simulink model "Hexa_CAD_ANSFT_Sim"  (R2024b)
settings: Solver=ode4  StartTime=0.0  StopTime=8  FixedStep=0.01  RelTol=1e-3
model workspace (MAT data in the model file):
  hover_2m = [0  0  0  0  0  0; 0  0  0  0  0  0; 2  2  2  2  2  2; 0  0  0  0  0  0; 0  0  0  0  0  0; 0  0  0  0  0  0]
  square = [0  0  0  0  0  0; 0  0  0  0  0  0; 2.5  2.5  2.5  2.5  2.5  0; 0  0  0  0  0  0; 0  0  0  0  0  0; 0  0  0  0  0  0]
  tf = Simulink.Parameter
  tf.Value = 60
  tf.Complexity = 'real'
  tf.Dimensions = [1 1]
  tf.DataType = 'auto'
  tray0 = [0  0.2  0  0  0  0; 0  0.15  0  0  0  0; 0  2  2  2  2  0; 0  0  0  0  0  0; 0  0  0  0  0  0; 0  0  0  0  0  0]
  tray1 = [0  0  0  0  0  0; 0  0  0  0  0  0; 0  5  2.5  5  2.5  0; 0  0  0  0  0  0; 0  0  0  0  0  0; 0  0  0  0  0  0]
  tray2 = [0  2  2  -2  -2  0; 0  0  -2  -2  2  0; 0  5  2.5  5  2.5  0; 0  0  0  0  0  0; 0  0  0  0  0  0; 0  0  0  0  0  0]
  tray3 = [0  2  2  -2  -2  0; 0  0  -2  -2  2  0; 0  5  2.5  5  2.5  0; 0  0  0  0  0  0; 0  0  0  0  0  0; 0  0  0.785  1.042  0.785  0]
  tray4 = [0  2  2  -2  -2  0; 0  0  -2  -2  2  0; 0  5  2.5  5  2.5  0; 0  0.15  0.15  0.15  0.15  0; 0  0  0  0  0  0; 0  0  0.785  1.57  0.785  0]
  tray5 = [0  0  0  0  0  0; 0  0  0  0  0  0; 0  5  2.5  5  2.5  0; 0  0.15  0.15  0  0  0; 0  0  0.15  0.15  0  0; 0  0  0  0  0  0]
  tray_yaw = [0  0  0  0  0  0; 0  0  0  0  0  0; 0  5  2.5  5  2.5  0; 0  0  0  0  0  0; 0  0  0  0  0  0; 0  0  0.785  1.57  0.785  0]
undefined symbols (not defined in the file or in its folder): F, Light, MIL, smiData, X, Y, Z
libraries: sm_lib x238, nesl_utility x29, dspobslib x7, simulink x3, sharedtransform x2, robotcorelib x1, aerolibwind2 x1
(part 1 of 6)
settings Model: Creator=Jorge  LastModifiedBy=danyy
settings DataIOCC: ReturnWorkspaceOutputs=off
settings OptimizationCC: ReuseModelBlockBuffer=off
settings DebuggingCC: UnconnectedInputMsg=warning  UnconnectedOutputMsg=warning  UnconnectedLineMsg=warning
settings ModelReferenceCC: EnableRefExpFcnMdlSchedulingChecks=on
settings RTWCC: GPUComputeCapability=3.5  DLArmComputeVersion=19.05

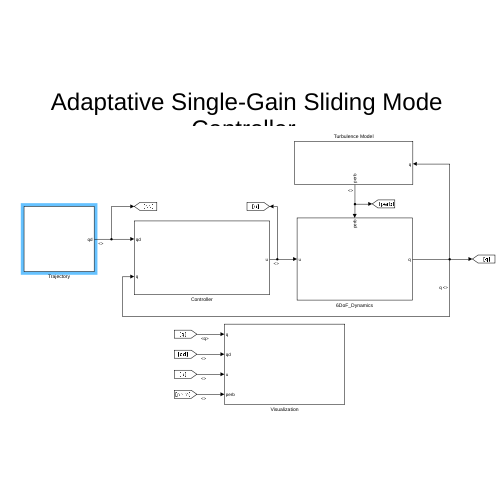
[thumbnail: Simulink's stored preview of the top-level diagram]
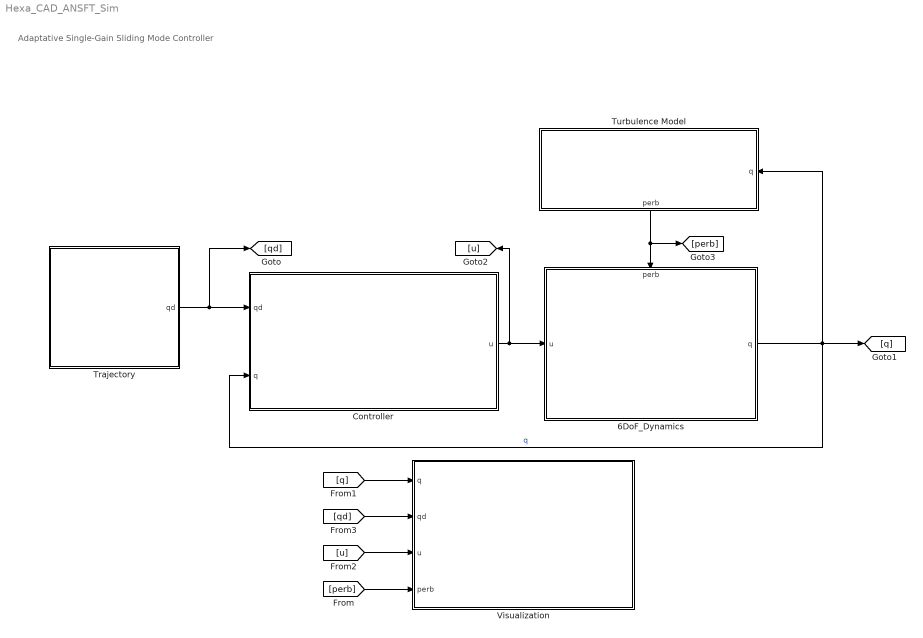
== system Hexa_CAD_ANSFT_Sim ==
  note: Adaptative Single-Gain Sliding Mode Controller
  6DoF_Dynamics : Subsystem
      settings: PortSchema="{\"entries\":[{\"content\":{\"sides\":[{\"content\":{\"connectorIds\":[\"In1\"]},\"type\":\"ConnectorPlacement.EquallySpacedRectSide\",\"uuid\":\"d79ec49c-5563-41e0-ac59-6e897bc19fda\"},{\"content\":{\"connectorIds\":[\"Out1\"],\"side\":\"RIGHT\"},\"type\":\"ConnectorPlacement.EquallySpacedRectSide\",\"uuid\":\"1255043e-c90e-4bae-9fb4-4fa06f36f53e\"},{\"content\":{\"connectorIds\":[\"In2\"],\"side\":\"TOP\"},\"type\":\"ConnectorPlacement.EquallySpacedRectSide\",\"uuid\":\"823ada36-3f22-4ee3-87a1-180276f622bc\"}]},\"type\":\"ConnectorPlacement.EquallySpacedConnector\",\"uuid\":\"7403b609-b333-4977-a854-ed7a71f74338\"}],\"packageUris\":[\"http://schema.mathworks.com/mf0/Connector/R2020b\"],\"version\":\"1.0\"}"
  Controller : Subsystem
  Trajectory : Subsystem
  Turbulence Model : Subsystem
      settings: PortSchema="{\"entries\":[{\"content\":{\"sides\":[{\"content\":{},\"type\":\"ConnectorPlacement.EquallySpacedRectSide\",\"uuid\":\"f78b09a1-2be7-4ada-a431-40e3e9754158\"},{\"content\":{\"connectorIds\":[\"In1\"],\"side\":\"RIGHT\"},\"type\":\"ConnectorPlacement.EquallySpacedRectSide\",\"uuid\":\"90af6136-accc-442b-9679-ef2510f8cfdd\"},{\"content\":{\"side\":\"TOP\"},\"type\":\"ConnectorPlacement.EquallySpacedRectSide\",\"uuid\":\"ed3143b1-02fd-44b4-8f22-c95c41bbcf7f\"},{\"content\":{\"connectorIds\":[\"Out1\"],\"side\":\"BOTTOM\"},\"type\":\"ConnectorPlacement.EquallySpacedRectSide\",\"uuid\":\"715dd93d-905b-40a3-aeb3-61c6c8d9767d\"}]},\"type\":\"ConnectorPlacement.EquallySpacedConnector\",\"uuid\":\"95dc4bc2-a941-4378-8d0a-e3a54b47d1ac\"}],\"packageUris\":[\"http://schema.mathworks.com/mf0/Connector/R2020b\"],\"version\":\"1.0\"}"
  Visualization : Subsystem
  wires:
  Trajectory/1(qd) -> [qd], Controller/1(qd)
  Controller/1(u) -> [u], 6DoF_Dynamics/1(u)
  6DoF_Dynamics/1(q) -> Turbulence Model/1(q), [q], Controller/2(q)  "q"
  Turbulence Model/1(perb) -> 6DoF_Dynamics/2(perb), [perb]
  [q] -> Visualization/1(q)
  [qd] -> Visualization/2(qd)
  [perb] -> Visualization/4(perb)
  [u] -> Visualization/3(u)

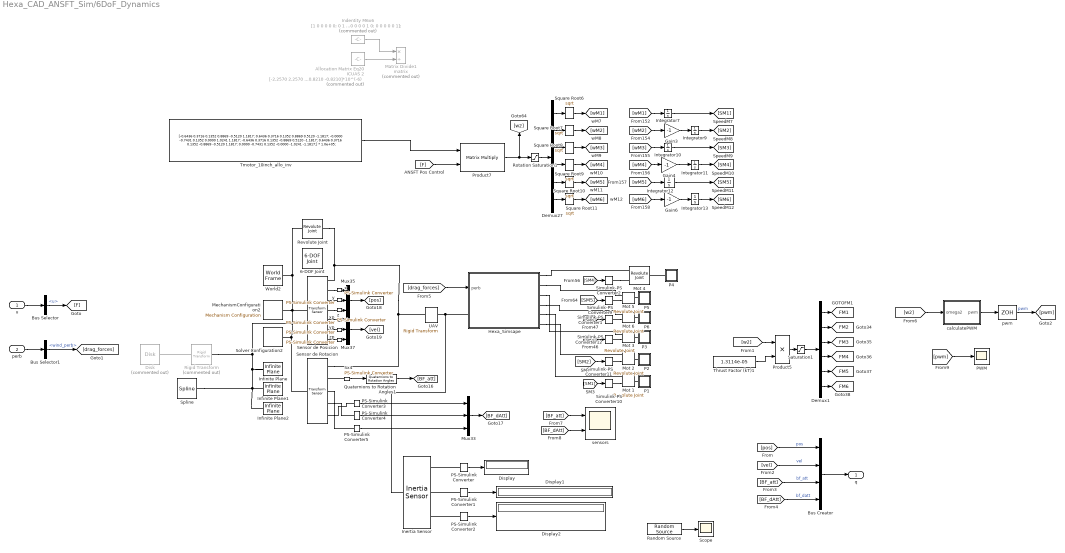
== system Hexa_CAD_ANSFT_Sim/6DoF_Dynamics ==
  u : Inport
  perb : Inport  Port=2
  6-DOF Joint : sm_lib/Joints/6-DOF Joint  JointMode=Normal  CompositeWrenchDir=FollowerOnBase  CompositeWrenchFrame=BaseFrame  SenseConstraintForce=off  SenseConstraintTorque=off  SenseTotalForce=off  SenseTotalTorque=off  PxPositionTargetSpecify=off  PxPositionTargetPriority=High  PxPositionTargetValue=0  PxPositionTargetValueUnits=m  PxVelocityTargetSpecify=off  PxVelocityTargetPriority=High  PxVelocityTargetValue=0  PxVelocityTargetValueUnits=m/s  PxEquilibriumPosition=0  PxEquilibriumPositionUnits=m  PxSpringStiffness=0  PxSpringStiffnessUnits=N/m  PxDampingCoefficient=0  PxDampingCoefficientUnits=N/(m/s)  PxLowerLimitSpecify=off  PxLowerLimitBound=-1  PxLowerLimitBoundUnits=m  PxLowerLimitStiffness=1e6  PxLowerLimitStiffnessUnits=N/m  PxLowerLimitDamping=1e3  PxLowerLimitDampingUnits=N/(m/s)  PxLowerLimitTransitionRegionWidth=1e-4  PxLowerLimitTransitionRegionWidthUnits=m  PxUpperLimitSpecify=off  PxUpperLimitBound=1  PxUpperLimitBoundUnits=m  PxUpperLimitStiffness=1e6  PxUpperLimitStiffnessUnits=N/m  PxUpperLimitDamping=1e3  PxUpperLimitDampingUnits=N/(m/s)  PxUpperLimitTransitionRegionWidth=1e-4  PxUpperLimitTransitionRegionWidthUnits=m  PxTorqueActuationMode=NoTorque  PxMotionActuationMode=ComputedMotion  PxSensePosition=off  PxSenseVelocity=off  PxSenseAcceleration=off  PxSenseTorqueForce=off  PxSenseLowerLimitTorqueForce=off  PxSenseUpperLimitTorqueForce=off  PyPositionTargetSpecify=off  PyPositionTargetPriority=High  PyPositionTargetValue=0  PyPositionTargetValueUnits=m  PyVelocityTargetSpecify=off  PyVelocityTargetPriority=High  PyVelocityTargetValue=0  PyVelocityTargetValueUnits=m/s  PyEquilibriumPosition=0  PyEquilibriumPositionUnits=m  PySpringStiffness=0  PySpringStiffnessUnits=N/m  PyDampingCoefficient=0  PyDampingCoefficientUnits=N/(m/s)  PyLowerLimitSpecify=off  PyLowerLimitBound=-1  PyLowerLimitBoundUnits=m  PyLowerLimitStiffness=1e6  PyLowerLimitStiffnessUnits=N/m  PyLowerLimitDamping=1e3  PyLowerLimitDampingUnits=N/(m/s)  PyLowerLimitTransitionRegionWidth=1e-4  PyLowerLimitTransitionRegionWidthUnits=m  PyUpperLimitSpecify=off  PyUpperLimitBound=1  PyUpperLimitBoundUnits=m  PyUpperLimitStiffness=1e6  PyUpperLimitStiffnessUnits=N/m  PyUpperLimitDamping=1e3  PyUpperLimitDampingUnits=N/(m/s)  PyUpperLimitTransitionRegionWidth=1e-4  PyUpperLimitTransitionRegionWidthUnits=m  PyTorqueActuationMode=NoTorque  PyMotionActuationMode=ComputedMotion  PySensePosition=off  PySenseVelocity=off  PySenseAcceleration=off  PySenseTorqueForce=off  PySenseLowerLimitTorqueForce=off  PySenseUpperLimitTorqueForce=off  PzPositionTargetSpecify=on  PzPositionTargetPriority=High  PzPositionTargetValue=0.20  PzPositionTargetValueUnits=m  PzVelocityTargetSpecify=off  PzVelocityTargetPriority=High  PzVelocityTargetValue=0  PzVelocityTargetValueUnits=m/s  PzEquilibriumPosition=0  PzEquilibriumPositionUnits=m  PzSpringStiffness=0  PzSpringStiffnessUnits=N/m  PzDampingCoefficient=0  PzDampingCoefficientUnits=N/(m/s)  PzLowerLimitSpecify=off  PzLowerLimitBound=-1  PzLowerLimitBoundUnits=m  PzLowerLimitStiffness=1e6  PzLowerLimitStiffnessUnits=N/m  PzLowerLimitDamping=1e3  PzLowerLimitDampingUnits=N/(m/s)  PzLowerLimitTransitionRegionWidth=1e-4  PzLowerLimitTransitionRegionWidthUnits=m  PzUpperLimitSpecify=off  PzUpperLimitBound=1  PzUpperLimitBoundUnits=m  PzUpperLimitStiffness=1e6  PzUpperLimitStiffnessUnits=N/m  PzUpperLimitDamping=1e3  PzUpperLimitDampingUnits=N/(m/s)  PzUpperLimitTransitionRegionWidth=1e-4  PzUpperLimitTransitionRegionWidthUnits=m  PzTorqueActuationMode=NoTorque  PzMotionActuationMode=ComputedMotion  PzSensePosition=off  PzSenseVelocity=off  PzSenseAcceleration=off  PzSenseTorqueForce=off  PzSenseLowerLimitTorqueForce=off  PzSenseUpperLimitTorqueForce=off  SphPositionTargetSpecify=off  SphPositionTargetPriority=High  SphPositionTargetRotationMethod=StandardAxis  SphPositionTargetFollAlignAxisA=+X  SphPositionTargetBaseAlignAxisA=+Y  SphPositionTargetFollAlignAxisB=+Y  SphPositionTargetBaseAlignAxisB=+Z  SphPositionTargetRotationStandardAxis=+Z  SphPositionTargetRotationAngle=-45  SphPositionTargetRotationAngleUnits=deg  SphPositionTargetRotationArbitraryAxis=[0 0 1]  SphPositionTargetRotationSequenceAxes=FollowerAxes  SphPositionTargetRotationSequence=XYX  SphPositionTargetRotationSequenceAngles=[0 0 0]  SphPositionTargetRotationSequenceAnglesUnits=deg  SphPositionTargetRotationMatrix=[1 0 0; 0 1 0; 0 0 1]  SphPositionTargetQuaternion=[1 0 0 0]  SphVelocityTargetSpecify=off  SphVelocityTargetPriority=High  SphVelocityTargetValue=[0 0 0]  SphVelocityTargetValueUnits=deg/s  SphVelocityTargetInFollowerFrame=on  SphEqPosRotationMethod=None  SphEqPosFollAlignAxisA=+X  SphEqPosBaseAlignAxisA=+Y  SphEqPosFollAlignAxisB=+Y  SphEqPosBaseAlignAxisB=+Z  SphEqPosRotationStandardAxis=+Z  SphEqPosRotationAngle=0.0  SphEqPosRotationAngleUnits=deg  SphEqPosRotationArbitraryAxis=[0 0 1]  SphEqPosRotationSequenceAxes=FollowerAxes  SphEqPosRotationSequence=XYX  SphEqPosRotationSequenceAngles=[0 0 0]  SphEqPosRotationSequenceAnglesUnits=deg  SphEqPosRotationMatrix=[1 0 0; 0 1 0; 0 0 1]  SphEqPosQuaternion=[1 0 0 0]  SphSpringStiffness=0  SphSpringStiffnessUnits=N*m/deg  SphDampingCoefficient=0  SphDampingCoefficientUnits=N*m/(deg/s)  SphLowerLimitSpecify=off  SphLowerLimitBound=15  SphLowerLimitBoundUnits=deg  SphLowerLimitStiffness=1e4  SphLowerLimitStiffnessUnits=N*m/deg  SphLowerLimitDamping=10  SphLowerLimitDampingUnits=N*m/(deg/s)  SphLowerLimitTransitionRegionWidth=0.1  SphLowerLimitTransitionRegionWidthUnits=deg  SphUpperLimitSpecify=off  SphUpperLimitBound=45  SphUpperLimitBoundUnits=deg  SphUpperLimitStiffness=1e4  SphUpperLimitStiffnessUnits=N*m/deg  SphUpperLimitDamping=10  SphUpperLimitDampingUnits=N*m/(deg/s)  SphUpperLimitTransitionRegionWidth=0.1  SphUpperLimitTransitionRegionWidthUnits=deg  SphTorqueActuationMode=NoTorque  SphActuateTorqueX=off  SphActuateTorqueY=off  SphActuateTorqueZ=off  SphActuateTorque=off  SphActuationFrame=BaseFrame  SphSensePosition=off  SphSenseVelocityX=off  SphSenseVelocityY=off  SphSenseVelocityZ=off  SphSenseVelocity=off  SphSenseAccelerationX=off  SphSenseAccelerationY=off  SphSenseAccelerationZ=off  SphSenseAcceleration=off  SphSenseLowerLimitTorqueMag=off  SphSenseUpperLimitTorqueMag=off  SphSensingFrame=BaseFrame
  Allocation Matrix Eq20 ICUAS 2 : Constant  Commented=on  Value=[-2.2570 2.2570 0 -2.2570 2.2570 0; 1.3030 1.3030 -2.6060 1.3030 1.3030 -2.6060; 7.160 7.160 7.160 7.160 7.160 7.160; 1.6370 1.6370 0 -1.6370 -1.6370 0; -0.945 0.945 1.891 0.945 -0.945 -1.891; 0.8210 -0.8210 0.8210 -0.8210 0.8210 -0.8210]*10^(-6)
  Bus Creator : BusCreator  Inputs=4
  Bus Selector : BusSelector  OutputSignals=u
  Bus Selector1 : BusSelector  OutputSignals=wind_perb
  Demux1 : Demux  Outputs=6
  Demux27 : Demux  Outputs=6
  Disk : sm_lib/Curves and Surfaces/Disk  Commented=on  Radius=5  RadiusUnits=m  GraphicType=FromGeometry  GraphicVisPropType=SimpleVisualProperties  GraphicDiffuseColor=[0.6353 0.07843 0.1843]  GraphicOpacity=0.8  GraphicSpecularColor=[0.5 0.5 0.5 1.0]  GraphicAmbientColor=[0.15 0.15 0.15 1.0]  GraphicEmissiveColor=[0.0 0.0 0.0 1.0]  GraphicShininess=75
  Display : Display
  Display1 : Display
  Display2 : Display
  Gain3 : Gain  Gain=-1
  Gain4 : Gain  Gain=-1
  Gain6 : Gain  Gain=-1
  Hexa_Simsape : Subsystem
  Indentity M6x6 : Constant  Commented=on  Value=[1 0 0 0 0 0; 0 1 0 0 0 0; 0 0 1 0 0 0; 0 0 0 1 0 0; 0 0 0 0 1 0; 0 0 0 0 0 1];
  Inertia Sensor : sm_lib/Body Elements/Inertia Sensor  SensorExtent=BodyGroup  SpanWeldJoints=off  ExcludeGroundedBodies=off  MeasurementFrame=Attached  SenseMass=on  SenseCenterOfMass=on  SenseInertiaMatrix=on  SenseCenteredInertiaMatrix=off  SensePrincipalInertiaMatrix=off  SenseRotationMatrix=off  GraphicType=PrincipalInertiaFrame  PrincipalInertiaFrameSize=20  GraphicVisPropType=SimpleVisualProperties  GraphicDiffuseColor=[0.5 0.5 0.5]  GraphicOpacity=1.0  GraphicSpecularColor=[0.5 0.5 0.5 1.0]  GraphicAmbientColor=[0.15 0.15 0.15 1.0]  GraphicEmissiveColor=[0.0 0.0 0.0 1.0]  GraphicShininess=75
  Infinite Plane : sm_lib/Curves and Surfaces/Infinite Plane  GraphicType=Rectangle  GraphicPlaneWidth=15  GraphicPlaneWidthUnits=m  GraphicPlaneHeight=15  GraphicPlaneHeightUnits=m  GraphicVisPropType=SimpleVisualProperties  GraphicDiffuseColor=[1 1 0.06667]  GraphicOpacity=0.25  GraphicSpecularColor=[1 1 1]  GraphicAmbientColor=[1 1 1]  GraphicEmissiveColor=[1 1 1]  GraphicShininess=75
  Infinite Plane1 : sm_lib/Curves and Surfaces/Infinite Plane  GraphicType=Rectangle  GraphicPlaneWidth=15  GraphicPlaneWidthUnits=m  GraphicPlaneHeight=0.01  GraphicPlaneHeightUnits=m  GraphicVisPropType=SimpleVisualProperties  GraphicDiffuseColor=[1 1 0.06667]  GraphicOpacity=0.5  GraphicSpecularColor=[0.5 0.5 0.5 1.0]  GraphicAmbientColor=[0.15 0.15 0.15 1.0]  GraphicEmissiveColor=[0.0 0.0 0.0 1.0]  GraphicShininess=75
  Infinite Plane2 : sm_lib/Curves and Surfaces/Infinite Plane  GraphicType=Rectangle  GraphicPlaneWidth=0.01  GraphicPlaneWidthUnits=m  GraphicPlaneHeight=15  GraphicPlaneHeightUnits=m  GraphicVisPropType=SimpleVisualProperties  GraphicDiffuseColor=[1 1 0.06667]  GraphicOpacity=0.5  GraphicSpecularColor=[0.5 0.5 0.5 1.0]  GraphicAmbientColor=[0.15 0.15 0.15 1.0]  GraphicEmissiveColor=[0.0 0.0 0.0 1.0]  GraphicShininess=75
  Integrator{7,9..13} (6 alike) : Integrator
  Matrix Divide1 : Product  Commented=on  Inputs=*/  Multiplication=Matrix(*)
  MechanismConfiguration2 : sm_lib/Utilities/Mechanism Configuration  UniformGravity=Constant  GravityVector=[0 0 -9.80665]  GravityVectorUnits=m/s^2  LinearizationDelta=0.01  JointModeTransitionNonlinearIterations=2
  Mot 1 : sm_lib/Joints/Revolute Joint  JointMode=Normal  CompositeWrenchDir=FollowerOnBase  CompositeWrenchFrame=BaseFrame  SenseConstraintForce=off  SenseConstraintTorque=off  SenseTotalForce=off  SenseTotalTorque=off  PositionTargetSpecify=on  PositionTargetPriority=Low  PositionTargetValue=smiData.RevoluteJoint(1).Rz.Pos  PositionTargetValueUnits=deg  VelocityTargetSpecify=off  VelocityTargetPriority=High  VelocityTargetValue=0  VelocityTargetValueUnits=deg/s  EquilibriumPosition=0  EquilibriumPositionUnits=deg  SpringStiffness=0  SpringStiffnessUnits=N*m/deg  DampingCoefficient=0  DampingCoefficientUnits=N*m/(deg/s)  LowerLimitSpecify=off  LowerLimitBound=-90  LowerLimitBoundUnits=deg  LowerLimitStiffness=1e4  LowerLimitStiffnessUnits=N*m/deg  LowerLimitDamping=10  LowerLimitDampingUnits=N*m/(deg/s)  LowerLimitTransitionRegionWidth=0.1  LowerLimitTransitionRegionWidthUnits=deg  UpperLimitSpecify=off  UpperLimitBound=90  UpperLimitBoundUnits=deg  UpperLimitStiffness=1e4  UpperLimitStiffnessUnits=N*m/deg  UpperLimitDamping=10  UpperLimitDampingUnits=N*m/(deg/s)  UpperLimitTransitionRegionWidth=0.1  UpperLimitTransitionRegionWidthUnits=deg  TorqueActuationMode=ComputedTorque  MotionActuationMode=InputMotion  SensePosition=off  SenseVelocity=off  SenseAcceleration=off  SenseTorqueForce=off  SenseLowerLimitTorqueForce=off  SenseUpperLimitTorqueForce=off
  Mot 2 : sm_lib/Joints/Revolute Joint  JointMode=Normal  CompositeWrenchDir=FollowerOnBase  CompositeWrenchFrame=BaseFrame  SenseConstraintForce=off  SenseConstraintTorque=off  SenseTotalForce=off  SenseTotalTorque=off  PositionTargetSpecify=on  PositionTargetPriority=Low  PositionTargetValue=smiData.RevoluteJoint(2).Rz.Pos  PositionTargetValueUnits=deg  VelocityTargetSpecify=off  VelocityTargetPriority=High  VelocityTargetValue=0  VelocityTargetValueUnits=deg/s  EquilibriumPosition=0  EquilibriumPositionUnits=deg  SpringStiffness=0  SpringStiffnessUnits=N*m/deg  DampingCoefficient=0  DampingCoefficientUnits=N*m/(deg/s)  LowerLimitSpecify=off  LowerLimitBound=-90  LowerLimitBoundUnits=deg  LowerLimitStiffness=1e4  LowerLimitStiffnessUnits=N*m/deg  LowerLimitDamping=10  LowerLimitDampingUnits=N*m/(deg/s)  LowerLimitTransitionRegionWidth=0.1  LowerLimitTransitionRegionWidthUnits=deg  UpperLimitSpecify=off  UpperLimitBound=90  UpperLimitBoundUnits=deg  UpperLimitStiffness=1e4  UpperLimitStiffnessUnits=N*m/deg  UpperLimitDamping=10  UpperLimitDampingUnits=N*m/(deg/s)  UpperLimitTransitionRegionWidth=0.1  UpperLimitTransitionRegionWidthUnits=deg  TorqueActuationMode=ComputedTorque  MotionActuationMode=InputMotion  SensePosition=off  SenseVelocity=off  SenseAcceleration=off  SenseTorqueForce=off  SenseLowerLimitTorqueForce=off  SenseUpperLimitTorqueForce=off
  Mot 3 : sm_lib/Joints/Revolute Joint  JointMode=Normal  CompositeWrenchDir=FollowerOnBase  CompositeWrenchFrame=BaseFrame  SenseConstraintForce=off  SenseConstraintTorque=off  SenseTotalForce=off  SenseTotalTorque=off  PositionTargetSpecify=on  PositionTargetPriority=Low  PositionTargetValue=smiData.RevoluteJoint(3).Rz.Pos  PositionTargetValueUnits=deg  VelocityTargetSpecify=off  VelocityTargetPriority=High  VelocityTargetValue=0  VelocityTargetValueUnits=deg/s  EquilibriumPosition=0  EquilibriumPositionUnits=deg  SpringStiffness=0  SpringStiffnessUnits=N*m/deg  DampingCoefficient=0  DampingCoefficientUnits=N*m/(deg/s)  LowerLimitSpecify=off  LowerLimitBound=-90  LowerLimitBoundUnits=deg  LowerLimitStiffness=1e4  LowerLimitStiffnessUnits=N*m/deg  LowerLimitDamping=10  LowerLimitDampingUnits=N*m/(deg/s)  LowerLimitTransitionRegionWidth=0.1  LowerLimitTransitionRegionWidthUnits=deg  UpperLimitSpecify=off  UpperLimitBound=90  UpperLimitBoundUnits=deg  UpperLimitStiffness=1e4  UpperLimitStiffnessUnits=N*m/deg  UpperLimitDamping=10  UpperLimitDampingUnits=N*m/(deg/s)  UpperLimitTransitionRegionWidth=0.1  UpperLimitTransitionRegionWidthUnits=deg  TorqueActuationMode=ComputedTorque  MotionActuationMode=InputMotion  SensePosition=off  SenseVelocity=off  SenseAcceleration=off  SenseTorqueForce=off  SenseLowerLimitTorqueForce=off  SenseUpperLimitTorqueForce=off
  Mot 4 : sm_lib/Joints/Revolute Joint  JointMode=Normal  CompositeWrenchDir=FollowerOnBase  CompositeWrenchFrame=BaseFrame  SenseConstraintForce=off  SenseConstraintTorque=off  SenseTotalForce=off  SenseTotalTorque=off  PositionTargetSpecify=on  PositionTargetPriority=Low  PositionTargetValue=smiData.RevoluteJoint(5).Rz.Pos  PositionTargetValueUnits=deg  VelocityTargetSpecify=off  VelocityTargetPriority=High  VelocityTargetValue=0  VelocityTargetValueUnits=deg/s  EquilibriumPosition=0  EquilibriumPositionUnits=deg  SpringStiffness=0  SpringStiffnessUnits=N*m/deg  DampingCoefficient=0  DampingCoefficientUnits=N*m/(deg/s)  LowerLimitSpecify=off  LowerLimitBound=-90  LowerLimitBoundUnits=deg  LowerLimitStiffness=1e4  LowerLimitStiffnessUnits=N*m/deg  LowerLimitDamping=10  LowerLimitDampingUnits=N*m/(deg/s)  LowerLimitTransitionRegionWidth=0.1  LowerLimitTransitionRegionWidthUnits=deg  UpperLimitSpecify=off  UpperLimitBound=90  UpperLimitBoundUnits=deg  UpperLimitStiffness=1e4  UpperLimitStiffnessUnits=N*m/deg  UpperLimitDamping=10  UpperLimitDampingUnits=N*m/(deg/s)  UpperLimitTransitionRegionWidth=0.1  UpperLimitTransitionRegionWidthUnits=deg  TorqueActuationMode=ComputedTorque  MotionActuationMode=InputMotion  SensePosition=off  SenseVelocity=off  SenseAcceleration=off  SenseTorqueForce=off  SenseLowerLimitTorqueForce=off  SenseUpperLimitTorqueForce=off
  Mot 5 : sm_lib/Joints/Revolute Joint  JointMode=Normal  CompositeWrenchDir=FollowerOnBase  CompositeWrenchFrame=BaseFrame  SenseConstraintForce=off  SenseConstraintTorque=off  SenseTotalForce=off  SenseTotalTorque=off  PositionTargetSpecify=on  PositionTargetPriority=Low  PositionTargetValue=smiData.RevoluteJoint(6).Rz.Pos  PositionTargetValueUnits=deg  VelocityTargetSpecify=off  VelocityTargetPriority=High  VelocityTargetValue=0  VelocityTargetValueUnits=deg/s  EquilibriumPosition=0  EquilibriumPositionUnits=deg  SpringStiffness=0  SpringStiffnessUnits=N*m/deg  DampingCoefficient=0  DampingCoefficientUnits=N*m/(deg/s)  LowerLimitSpecify=off  LowerLimitBound=-90  LowerLimitBoundUnits=deg  LowerLimitStiffness=1e4  LowerLimitStiffnessUnits=N*m/deg  LowerLimitDamping=10  LowerLimitDampingUnits=N*m/(deg/s)  LowerLimitTransitionRegionWidth=0.1  LowerLimitTransitionRegionWidthUnits=deg  UpperLimitSpecify=off  UpperLimitBound=90  UpperLimitBoundUnits=deg  UpperLimitStiffness=1e4  UpperLimitStiffnessUnits=N*m/deg  UpperLimitDamping=10  UpperLimitDampingUnits=N*m/(deg/s)  UpperLimitTransitionRegionWidth=0.1  UpperLimitTransitionRegionWidthUnits=deg  TorqueActuationMode=ComputedTorque  MotionActuationMode=InputMotion  SensePosition=off  SenseVelocity=off  SenseAcceleration=off  SenseTorqueForce=off  SenseLowerLimitTorqueForce=off  SenseUpperLimitTorqueForce=off
  Mot 6 : sm_lib/Joints/Revolute Joint  JointMode=Normal  CompositeWrenchDir=FollowerOnBase  CompositeWrenchFrame=BaseFrame  SenseConstraintForce=off  SenseConstraintTorque=off  SenseTotalForce=off  SenseTotalTorque=off  PositionTargetSpecify=on  PositionTargetPriority=Low  PositionTargetValue=smiData.RevoluteJoint(4).Rz.Pos  PositionTargetValueUnits=deg  VelocityTargetSpecify=off  VelocityTargetPriority=High  VelocityTargetValue=0  VelocityTargetValueUnits=deg/s  EquilibriumPosition=0  EquilibriumPositionUnits=deg  SpringStiffness=0  SpringStiffnessUnits=N*m/deg  DampingCoefficient=0  DampingCoefficientUnits=N*m/(deg/s)  LowerLimitSpecify=off  LowerLimitBound=-90  LowerLimitBoundUnits=deg  LowerLimitStiffness=1e4  LowerLimitStiffnessUnits=N*m/deg  LowerLimitDamping=10  LowerLimitDampingUnits=N*m/(deg/s)  LowerLimitTransitionRegionWidth=0.1  LowerLimitTransitionRegionWidthUnits=deg  UpperLimitSpecify=off  UpperLimitBound=90  UpperLimitBoundUnits=deg  UpperLimitStiffness=1e4  UpperLimitStiffnessUnits=N*m/deg  UpperLimitDamping=10  UpperLimitDampingUnits=N*m/(deg/s)  UpperLimitTransitionRegionWidth=0.1  UpperLimitTransitionRegionWidthUnits=deg  TorqueActuationMode=ComputedTorque  MotionActuationMode=InputMotion  SensePosition=off  SenseVelocity=off  SenseAcceleration=off  SenseTorqueForce=off  SenseLowerLimitTorqueForce=off  SenseUpperLimitTorqueForce=off
  Mux33 : Mux  Inputs=3
  Mux35 : Mux  Inputs=3
  Mux37 : Mux  Inputs=3
  P1 : Subsystem
  P2 : Subsystem
  P3 : Subsystem
  P4 : Subsystem
  P5 : Subsystem
  P6 : Subsystem
  PS-Simulink Converter : nesl_utility/PS-Simulink Converter  PhysicalDomain=network_engine_domain  SubClassName=ps_output  LeftPortType=input  RightPortType=output  PseudoPeriodic=off  Frequencies=[]  VectorFormat=inherit  Unit=inherit  AffineConversion=off
  PS-Simulink Converter1 : nesl_utility/PS-Simulink Converter  PhysicalDomain=network_engine_domain  SubClassName=ps_output  LeftPortType=input  RightPortType=output  PseudoPeriodic=off  Frequencies=[]  VectorFormat=inherit  Unit=inherit  AffineConversion=off
  PS-Simulink Converter2 : nesl_utility/PS-Simulink Converter  PhysicalDomain=network_engine_domain  SubClassName=ps_output  LeftPortType=input  RightPortType=output  PseudoPeriodic=off  Frequencies=[]  VectorFormat=inherit  Unit=inherit  AffineConversion=off
  PS-Simulink Converter3 : nesl_utility/PS-Simulink Converter  PhysicalDomain=network_engine_domain  SubClassName=ps_output  LeftPortType=input  RightPortType=output  PseudoPeriodic=off  Frequencies=[]  VectorFormat=1-D array  Unit=inherit  AffineConversion=off
  PS-Simulink Converter4 : nesl_utility/PS-Simulink Converter  PhysicalDomain=network_engine_domain  SubClassName=ps_output  LeftPortType=input  RightPortType=output  PseudoPeriodic=off  Frequencies=[]  VectorFormat=1-D array  Unit=inherit  AffineConversion=off
  PS-Simulink Converter5 : nesl_utility/PS-Simulink Converter  PhysicalDomain=network_engine_domain  SubClassName=ps_output  LeftPortType=input  RightPortType=output  PseudoPeriodic=off  Frequencies=[]  VectorFormat=1-D array  Unit=inherit  AffineConversion=off
  PWM : Scope
  Product5 : Product
  Product7 : Product  Multiplication=Matrix(*)
  Quaternions to Rotation Angles1 : sharedtransform/Quaternions to Rotation Angles  rotationOrder=ZYX  aMode=aMode
  Random Source : dspobslib/Random Source  SrcType=Gaussian  NormMethod=Ziggurat  CltLength=12  MinVal=0  MaxVal=1  MeanVal=0.05  VarVal=0.001 * 0.001  RepMode=Not repeatable  rawSeed=1  IsInherit=off  SampMode=Discrete  SampTime=0.01  SampFrame=1  DataType=Double  OutComplex=Real  OutputFrames=off
  Revolute Joint : sm_lib/Joints/Revolute Joint  JointMode=Normal  CompositeWrenchDir=FollowerOnBase  CompositeWrenchFrame=BaseFrame  SenseConstraintForce=off  SenseConstraintTorque=off  SenseTotalForce=off  SenseTotalTorque=off  PositionTargetSpecify=on  PositionTargetPriority=High  PositionTargetValue=0  PositionTargetValueUnits=deg  VelocityTargetSpecify=off  VelocityTargetPriority=High  VelocityTargetValue=0  VelocityTargetValueUnits=deg/s  EquilibriumPosition=0  EquilibriumPositionUnits=deg  SpringStiffness=0  SpringStiffnessUnits=N*m/deg  DampingCoefficient=0  DampingCoefficientUnits=N*m/(deg/s)  LowerLimitSpecify=off  LowerLimitBound=-90  LowerLimitBoundUnits=deg  LowerLimitStiffness=1e4  LowerLimitStiffnessUnits=N*m/deg  LowerLimitDamping=10  LowerLimitDampingUnits=N*m/(deg/s)  LowerLimitTransitionRegionWidth=0.1  LowerLimitTransitionRegionWidthUnits=deg  UpperLimitSpecify=off  UpperLimitBound=90  UpperLimitBoundUnits=deg  UpperLimitStiffness=1e4  UpperLimitStiffnessUnits=N*m/deg  UpperLimitDamping=10  UpperLimitDampingUnits=N*m/(deg/s)  UpperLimitTransitionRegionWidth=0.1  UpperLimitTransitionRegionWidthUnits=deg  TorqueActuationMode=NoTorque  MotionActuationMode=ComputedMotion  SensePosition=off  SenseVelocity=off  SenseAcceleration=off  SenseTorqueForce=off  SenseLowerLimitTorqueForce=off  SenseUpperLimitTorqueForce=off
  Rigid Transform : sm_lib/Frames and Transforms/Rigid Transform  Commented=on  RotationMethod=None  FollAlignAxisA=+X  BaseAlignAxisA=+Y  FollAlignAxisB=+Y  BaseAlignAxisB=+Z  RotationStandardAxis=+Z  RotationAngle=0.0  RotationAngleUnits=deg  RotationArbitraryAxis=[0 0 1]  RotationSequenceAxes=FollowerAxes  RotationSequence=XYX  RotationSequenceAngles=[0 0 0]  RotationSequenceAnglesUnits=deg  RotationMatrix=[1 0 0; 0 1 0; 0 0 1]  Quaternion=[1 0 0 0]  TranslationMethod=Cartesian  TranslationCartesianOffset=[5 0 4]  TranslationCartesianOffsetUnits=m  TranslationStandardAxis=+Z  TranslationStandardOffset=0  TranslationStandardOffsetUnits=m  TranslationROffset=0  TranslationROffsetUnits=m  TranslationThetaOffset=0  TranslationThetaOffsetUnits=deg  TranslationZOffset=0  TranslationZOffsetUnits=m
  Rotation Saturation1 : Saturate  UpperLimit=1.4e6  LowerLimit=0
  Saturation1 : Saturate  UpperLimit=10  LowerLimit=0
  Scope : Scope
  Sensor de Posicion : sm_lib/Frames and Transforms/Transform Sensor  MeasurementFrame=World  RotationSequence=XYX  SenseAngle=off  SenseAxis=off  SenseQ=off  SenseR=off  SenseRotationSequence=off  SenseOmegaX=off  SenseOmegaY=off  SenseOmegaZ=off  SenseOmega=off  SenseQDot=off  SenseRDot=off  SenseRotationSequenceDot=off  SenseAlphaX=off  SenseAlphaY=off  SenseAlphaZ=off  SenseAlpha=off  SenseQDDot=off  SenseRDDot=off  SenseX=on  SenseY=on  SenseZ=on  SenseXYZ=off  SenseRad=off  SenseAzim=off  SenseDist=off  SenseInc=off  SenseXDot=on  SenseYDot=on  SenseZDot=on  SenseXYZDot=off  SenseRadDot=off  SenseAzimDot=off  SenseDistDot=off  SenseIncDot=off  SenseXDDot=off  SenseYDDot=off  SenseZDDot=off  SenseXYZDDot=off  SenseRadDDot=off  SenseAzimDDot=off  SenseDistDDot=off  SenseIncDDot=off
  Sensor de Rotacion : sm_lib/Frames and Transforms/Transform Sensor  MeasurementFrame=Follower  RotationSequence=XYX  SenseAngle=off  SenseAxis=off  SenseQ=on  SenseR=off  SenseRotationSequence=off  SenseOmegaX=on  SenseOmegaY=on  SenseOmegaZ=on  SenseOmega=off  SenseQDot=off  SenseRDot=off  SenseRotationSequenceDot=off  SenseAlphaX=off  SenseAlphaY=off  SenseAlphaZ=off  SenseAlpha=off  SenseQDDot=off  SenseRDDot=off  SenseX=off  SenseY=off  SenseZ=off  SenseXYZ=off  SenseRad=off  SenseAzim=off  SenseDist=off  SenseInc=off  SenseXDot=off  SenseYDot=off  SenseZDot=off  SenseXYZDot=off  SenseRadDot=off  SenseAzimDot=off  SenseDistDot=off  SenseIncDot=off  SenseXDDot=off  SenseYDDot=off  SenseZDDot=off  SenseXYZDDot=off  SenseRadDDot=off  SenseAzimDDot=off  SenseDistDDot=off  SenseIncDDot=off
  Simulink-PS Converter{1..2,9..12} (6 alike) : nesl_utility/Simulink-PS Converter  PhysicalDomain=network_engine_domain  SubClassName=ps_input  LeftPortType=input  RightPortType=output  PseudoPeriodic=off  Frequencies=[]  NoiseDistribution=none  NoiseParameters=[]  Unit=rad  AffineConversion=off  FilteringAndDerivatives=filter  SimscapeFilterOrder=2  InputFilterTimeConstant=0.01  UdotUserProvided=0
  Solver Configuration2 : nesl_utility/Solver Configuration  PhysicalDomain=network_engine_domain  SubClassName=solver  LeftPortType=input  RightPortType=generic  Tones=[]  Harmonics=[]  SimulateNoise=off  Profile=off  UseLocalSampling=off  EnableSwitchedLinearOptims=on  FrequencyDomain=off  UseCCode=off  RelTol=0.001  AbsTol=1e-06  MinStep=1e-09  ToWorkspace=off  RevertToSquareIcSolve=off  NumHomotopyIterations=100  PhasorMode=off  PhasorModeNumHarmonics=1  ConsistencySolver=NEWTON_FTOL  IndexReductionMethod=DerivativeReplacement  DoDC=off  ResidualTolerance=1e-09  ConsistencyTolSource=GLOBAL  ConsistencyAbsTol=0.001  ConsistencyRelTol=0.001  ConsistencyTolFactor=0.001  UseLocalSolver=off  LocalSolverChoice=NE_BACKWARD_EULER_ADVANCER  ResolveIndetEquations=on  FunctionEvalNumThread=1  LocalSolverSampleTime=0.01  DoFixedCost=off  MaxNonlinIter=3  MaxModeIter=2  ComputeImpulses=off  ImpulseIterations=2  LinearAlgebra=Full  LinearAlgebraNumThread=0  EquationFormulation=NE_TIME_EF  DelaysMemoryBudget=1024  AutomaticFiltering=on  FilteringTimeConstant=0.001  PartitionStorageMethod=AS_NEEDED  PartitionMemoryBudget=1024  PartitionMethod=ROBUST  MultibodyUseLocalSolver=off  MultibodyLocalSolverChoice=ODE1  MultibodyLocalSolverSampleTime=0.001
  Spline : sm_lib/Curves and Surfaces/Spline  DataPoints=[0 0 4; -5 5 4; -10 0 4; -5 -5 4]  DataPointsUnits=m  EndConditionType=Closed  GraphicType=FromGeometry  MarkerShape=Sphere  MarkerSize=10  GraphicVisPropType=SimpleVisualProperties  GraphicDiffuseColor=[0.6 0.0 0.0]  GraphicOpacity=1.0  GraphicSpecularColor=[0.5 0.5 0.5 1.0]  GraphicAmbientColor=[0.15 0.15 0.15 1.0]  GraphicEmissiveColor=[0.0 0.0 0.0 1.0]  GraphicShininess=75
  Square Root{6..11} (6 alike) : Sqrt
  Sx4 : nesl_utility/PS-Simulink Converter  PhysicalDomain=network_engine_domain  SubClassName=ps_output  LeftPortType=input  RightPortType=output  PseudoPeriodic=off  Frequencies=[]  VectorFormat=1-D array  Unit=inherit  AffineConversion=on
  Thrust Factor (kT)1 : Constant  Value=1.3114e-05
  Tmotor_10inch_allo_inv : Constant  Value=|
      | [-0.6436    0.3716    0.1352    0.8869   -0.5120    1.1817;
      |             0.6436    0.3716    0.1352    0.8869    0.5120   -1.1817;
      |             -0.0000   -0.7431    0.1352    0.0000    1.0241    1.1817;
      |             -0.6436    0.3716    0.1352   -0.8869    0.5120   -1.1817;
      |             0.6436    0.3716    0.1352   -0.8869   -0.5120    1.1817;
      |             0.0000   -0.7431    0.1352   -0.0000   -1.0241   -1.1817;] * 1.0e+05;
  UAV : sm_lib/Frames and Transforms/Rigid Transform  RotationMethod=RotationMatrix  FollAlignAxisA=+X  BaseAlignAxisA=+Y  FollAlignAxisB=+Y  BaseAlignAxisB=+Z  RotationStandardAxis=+Z  RotationAngle=0.0  RotationAngleUnits=deg  RotationArbitraryAxis=[0 0 1]  RotationSequenceAxes=FollowerAxes  RotationSequence=XYX  RotationSequenceAngles=[0 0 0]  RotationSequenceAnglesUnits=deg  RotationMatrix=[1 0 0; 0 1 0; 0 0 1]  Quaternion=[1 0 0 0]  TranslationMethod=Cartesian  TranslationCartesianOffset=[0.0195 0.01 -0.26]  TranslationCartesianOffsetUnits=m  TranslationStandardAxis=+Z  TranslationStandardOffset=-0.185  TranslationStandardOffsetUnits=m  TranslationROffset=0  TranslationROffsetUnits=m  TranslationThetaOffset=0  TranslationThetaOffsetUnits=deg  TranslationZOffset=0  TranslationZOffsetUnits=m
  World2 : sm_lib/Frames and Transforms/World Frame
  calculatePWM : MATLAB Function  TreatAsAtomicUnit=on
  pwm : ZeroOrderHold  SampleTime=-1
  sensors : Scope  NumInputPorts=2
  x : nesl_utility/PS-Simulink Converter  PhysicalDomain=network_engine_domain  SubClassName=ps_output  LeftPortType=input  RightPortType=output  PseudoPeriodic=off  Frequencies=[]  VectorFormat=1-D array  Unit=inherit  AffineConversion=on
  xp : nesl_utility/PS-Simulink Converter  PhysicalDomain=network_engine_domain  SubClassName=ps_output  LeftPortType=input  RightPortType=output  PseudoPeriodic=off  Frequencies=[]  VectorFormat=1-D array  Unit=inherit  AffineConversion=on
  y : nesl_utility/PS-Simulink Converter  PhysicalDomain=network_engine_domain  SubClassName=ps_output  LeftPortType=input  RightPortType=output  PseudoPeriodic=off  Frequencies=[]  VectorFormat=1-D array  Unit=inherit  AffineConversion=on
  yp : nesl_utility/PS-Simulink Converter  PhysicalDomain=network_engine_domain  SubClassName=ps_output  LeftPortType=input  RightPortType=output  PseudoPeriodic=off  Frequencies=[]  VectorFormat=1-D array  Unit=inherit  AffineConversion=on
  z : nesl_utility/PS-Simulink Converter  PhysicalDomain=network_engine_domain  SubClassName=ps_output  LeftPortType=input  RightPortType=output  PseudoPeriodic=off  Frequencies=[]  VectorFormat=1-D array  Unit=inherit  AffineConversion=on
  zp : nesl_utility/PS-Simulink Converter  PhysicalDomain=network_engine_domain  SubClassName=ps_output  LeftPortType=input  RightPortType=output  PseudoPeriodic=off  Frequencies=[]  VectorFormat=1-D array  Unit=inherit  AffineConversion=on
  q : Outport
  tag scope: FM1=global, FM2=global, FM3=global, FM4=global, FM5=global, FM6=global
  wires:
  Demux1/3 -> [FM3]
  Integrator13/1 -> [SM6]
  [w2] -> Product5/1
  Thrust Factor (kT)1/1 -> Product5/2
  Square Root8/1 -> [wM3]
  Square Root7/1 -> [wM2]
  [wM6] -> Gain6/1
  [wM1] -> Integrator7/1
  Square Root6/1 -> [wM1]
  Demux27/4 -> Square Root9/1
  Demux1/5 -> [FM5]
  [wM3] -> Integrator10/1
  Indentity M6x6/1 -> Matrix Divide1/1
  Quaternions to Rotation Angles1/1 -> [BF_att]
  Demux27/2 -> Square Root7/1
  Allocation Matrix Eq20 ICUAS 2/1 -> Matrix Divide1/2
  Gain3/1 -> Integrator9/1
  z/1 -> Mux35/3
  Square Root10/1 -> [wM5]
  yp/1 -> Mux37/2
  Product7/1 -> Rotation Saturation1/1, [w2]
  [SM4] -> Simulink-PS Converter2/1
  Rotation Saturation1/1 -> Demux27/1
  Demux1/1 -> [FM1]
  Gain6/1 -> Integrator13/1
  Integrator10/1 -> [SM3]
  Demux27/6 -> Square Root11/1
  [SM3] -> Simulink-PS Converter12/1
  x/1 -> Mux35/1
  [SM5] -> Simulink-PS Converter9/1
  Mux33/1 -> [BF_dAtt]
  Saturation1/1 -> Demux1/1
  PS-Simulink Converter3/1 -> Mux33/1
  Demux1/2 -> [FM2]
  Gain4/1 -> Integrator11/1
  Square Root9/1 -> [wM4]
  [SM2] -> Simulink-PS Converter11/1
  Square Root11/1 -> [wM6]
  [F] -> Product7/2
  Mux37/1 -> [vel]
  Sx4/1 -> Quaternions to Rotation Angles1/1
  Demux1/4 -> [FM4]
  Demux27/3 -> Square Root8/1
  Mux35/1 -> [pos]
  zp/1 -> Mux37/3
  Demux1/6 -> [FM6]
  [SM6] -> Simulink-PS Converter1/1
  Demux27/1 -> Square Root6/1
  Product5/1 -> Saturation1/1
  xp/1 -> Mux37/1
  Demux27/5 -> Square Root10/1
  [wM2] -> Gain3/1
  [wM5] -> Integrator12/1
  PS-Simulink Converter5/1 -> Mux33/3
  [wM4] -> Gain4/1
  PS-Simulink Converter4/1 -> Mux33/2
  y/1 -> Mux35/2
  [SM1] -> Simulink-PS Converter10/1
  u/1 -> Bus Selector/1
  Bus Selector/1 -> [F]  "<u>"
  [pos] -> Bus Creator/1  "pos"
  [vel] -> Bus Creator/2  "vel"
  [BF_att] -> Bus Creator/3  "bf_att"
  [BF_dAtt] -> Bus Creator/4  "bf_datt"
  Bus Creator/1 -> q/1
  perb/1 -> Bus Selector1/1
  Bus Selector1/1 -> [drag_forces]  "<wind_perb>"
  [drag_forces] -> Hexa_Simsape/1(perb)
  Tmotor_10inch_allo_inv/1 -> Product7/1
  [pwm] -> PWM/1
  pwm/1 -> [pwm]  "pwm"
  calculatePWM/1(pwm) -> pwm/1
  [w2] -> calculatePWM/1(omega2)
  Integrator12/1 -> [SM5]
  Integrator11/1 -> [SM4]
  Integrator7/1 -> [SM1]
  Integrator9/1 -> [SM2]
  Random Source/1 -> Scope/1
  PS-Simulink Converter/1 -> Display/1
  PS-Simulink Converter1/1 -> Display1/1
  PS-Simulink Converter2/1 -> Display2/1
  [BF_att] -> sensors/1
  [BF_dAtt] -> sensors/2
  connections:
  Simulink-PS Converter9/RConn1 -- Mot 5/LConn2
  P4/LConn1 -- Mot 4/RConn1
  Hexa_Simsape/RConn3 -- Mot 3/LConn1
  Hexa_Simsape/RConn6 -- Mot 2/LConn1
  Hexa_Simsape/RConn5 -- Mot 1/LConn1
  Simulink-PS Converter10/RConn1 -- Mot 1/LConn2
  Hexa_Simsape/RConn2 -- Mot 5/LConn1
  Sx4/LConn1 -- Sensor de Rotacion/RConn2
  Hexa_Simsape/RConn4 -- Mot 6/LConn1
  Simulink-PS Converter2/RConn1 -- Mot 4/LConn2
  P1/LConn1 -- Mot 1/RConn1
  P6/LConn1 -- Mot 6/RConn1
  y/LConn1 -- Sensor de Posicion/RConn3
  P2/LConn1 -- Mot 2/RConn1
  Hexa_Simsape/RConn1 -- Mot 4/LConn1
  Sensor de Rotacion/RConn4 -- PS-Simulink Converter4/LConn1
  Sensor de Posicion/RConn4 -- z/LConn1
  Sensor de Rotacion/RConn5 -- PS-Simulink Converter3/LConn1
  Sensor de Posicion/RConn6 -- yp/LConn1
  P3/LConn1 -- Mot 3/RConn1
  Sensor de Rotacion/RConn3 -- PS-Simulink Converter5/LConn1
  Sensor de Posicion/RConn7 -- zp/LConn1
  Sensor de Rotacion/RConn1 -- Revolute Joint/RConn1 -- Sensor de Posicion/RConn1 -- UAV/LConn1
  Simulink-PS Converter11/RConn1 -- Mot 2/LConn2
  Sensor de Rotacion/LConn1 -- Spline/LConn1 -- Infinite Plane2/LConn1 -- Infinite Plane1/LConn1 -- Infinite Plane/LConn1 -- Rigid Transform/RConn1 -- Sensor de Posicion/LConn1 -- MechanismConfiguration2/RConn1 -- Revolute Joint/LConn1 -- World2/RConn1 -- Solver Configuration2/RConn1
  Simulink-PS Converter12/RConn1 -- Mot 3/LConn2
  Sensor de Posicion/RConn2 -- x/LConn1
  P5/LConn1 -- Mot 5/RConn1
  Sensor de Posicion/RConn5 -- xp/LConn1
  UAV/RConn1 -- Inertia Sensor/LConn1 -- Hexa_Simsape/LConn1
  Simulink-PS Converter1/RConn1 -- Mot 6/LConn2
  Rigid Transform/LConn1 -- Disk/LConn1
  PS-Simulink Converter2/LConn1 -- Inertia Sensor/RConn3
  PS-Simulink Converter1/LConn1 -- Inertia Sensor/RConn2
  PS-Simulink Converter/LConn1 -- Inertia Sensor/RConn1

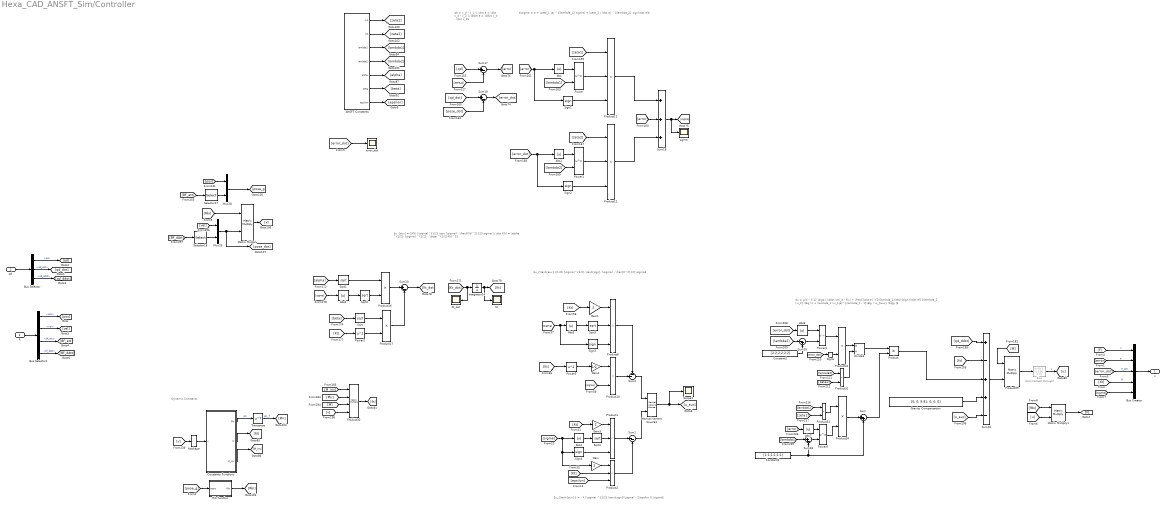
== system Hexa_CAD_ANSFT_Sim/Controller ==
  note: $u = g(x)^{-1} \bigg [ \ddot \chi_d - f(x) + \frac{|\dot e|^{2-\lambda_2}\text{sign}(\dot e)}{\lambda_2 \xi_2} \Big (1 + \lambda_1 \xi_1|e|^{\lambda_1 - 1}\Big ) -u_{aux} \bigg ]$
  note: $e = x_d - x_1 \\ \dot e = \dot x_d - x_2 \\ \ddot e = \ddot x_d - \dot x_2$
  note: $\sigma = e + \zeta_1 |e| ^{\lambda_1} sign(e) + \zeta_2 | \dot e| ^{\lambda_2} sign(\dot e)$
  note: $u_{aux}=-2K(t) |\sigma|^{1/2} sign (\sigma) - \frac{K(t)^2}{2}\sigma \\ \dot K(t) = \alpha ^{1/2} |\sigma| ^{1/2} - \beta ^{1/2}K(t)^2$
  note: Dynamic Constants
  note: $u_{\text{aux}}=-2K |\sigma|^{1/2} \text{sign} (\sigma) - \frac{K^2}{2}\sigma$
  note: $u_{\text{aux}} = - K |\sigma| ^{1/2} \text{sign}(\sigma) - 2\epsilon K \sigma$
  qd : Inport
  q : Inport  Port=2
  ANSFT Constants : MATLAB Function  TreatAsAtomicUnit=on
  Abs{,1..4,6..7} (7 alike) : Abs  SaturateOnIntegerOverflow=off
  Bias : Bias  Commented=through  Bias=[0; 0; 0; 0.08; 0; 0]  SaturateOnIntegerOverflow=off
  Bus Creator : BusCreator  Inputs=5
  Bus Selector : BusSelector  OutputSignals=qd,qd_dot,qd_ddot
  Bus Selector1 : BusSelector  OutputSignals=pos,vel,bf_att,bf_datt
  Constant2 : Constant  Value=[2;2;2;2;2;2]
  Constant3 : Constant  Value=[1;1;1;1;1;1]
  Constants Functions : MATLAB Function  TreatAsAtomicUnit=on
  Divide3 : Product  Inputs=*/
  Gain : Gain  Gain=2
  Gain1 : Gain  Gain=2
  Gain2 : Gain  Gain=1/2
  Gain3 : Gain  Gain=2
  Gravity Compensation : Constant  Value=[0; 0; 9.81; 0; 0; 0]
  Integrator14 : Integrator  InitialCondition=[0;0;0;0;0;0]
  Kt : Scope
  Kt_dot : Scope
  Manual Variant Source3 : simulink/Signal Routing/Manual Variant Source  NumChoices=2  LabelModeActiveChoice=V_2
  Matrix Multiply : Product  Multiplication=Matrix(*)
  Matrix Multiply1 : Product  Multiplication=Matrix(*)
  Mux28 : Mux  Inputs=2
  Mux29 : Mux  Inputs=2
  Power{,1,4..5} (4 alike) : Math  Operator=pow
  Power2 : Math  Operator=square
  Power3 : Math  Operator=square
  Product{,10,16..17,31..34} (8 alike) : Product
  Product{1..2,8,11..12} (5 alike) : Product  Inputs=3
  Product29 : Product  Multiplication=Matrix(*)
  Product30 : Product  Inputs=4  Multiplication=Matrix(*)
  Reshape : Reshape  OutputDimensionality=Customize  OutputDimensions=[6,1]
  Rib function : MATLAB Function  TreatAsAtomicUnit=on
  Scope1 : Scope
  Selector17 : Selector  InputPortWidth=3  IndexOptions=Index vector (dialog)  Indices=[3 2 1]  OutputSizes=1
  Selector18 : Selector  InputPortWidth=3  IndexOptions=Index vector (dialog)  Indices=[3 2 1]  OutputSizes=1
  Sign{1..4,6} (5 alike) : Signum
  Sqrt{,1..4} (5 alike) : Sqrt
  Sum : Sum  Inputs=|++
  Sum1 : Sum  Inputs=|--
  Sum{17,19..20,28} (4 alike) : Sum  Inputs=|+-
  Sum18 : Sum  Inputs=+++
  Sum23 : Sum  Inputs=+-++-
  Sum26 : Sum  Inputs=|-+
  Sum4 : Sum  Inputs=--|
  Transpose : Math  Operator=transpose
  error_dot : Scope
  sigma : Scope
  u : Outport
  wires:
  [zeta2] -> Product12/1
  [lambda1] -> Power/2
  Abs1/1 -> Power1/1
  [pose_g] -> Sum17/2
  Power5/1 -> Product34/2
  ANSFT Constants/4(lambda2) -> [lambda2]
  [Phi] -> Product30/2
  Product17/1 -> Sum20/2
  [v] -> Product30/4
  Sum20/1 -> [Kt_dot]
  [zeta2] -> Product32/2
  Sum19/1 -> [error_dot]
  Power4/1 -> Product31/1
  [error] -> Abs7/1
  [M_inv] -> Product30/1
  Product11/1 -> Sum18/1
  [lambda2] -> Power1/2
  [error_dot] -> Sign6/1
  [u_aux] -> Sum23/5
  Sign2/1 -> Product12/3
  Gravity Compensation/1 -> Sum23/4
  ANSFT Constants/6(beta) -> [beta]
  [lambda1] -> Sum28/1
  Sum28/1 -> Power5/2
  Product12/1 -> Sum18/3
  [alpha] -> Sqrt1/1
  Product/1 -> Sum23/3
  Power2/1 -> Product17/2
  [M] -> Product29/1
  [beta] -> Sqrt/1
  [sigma] -> Abs2/1
  [fx] -> Sum23/2
  ANSFT Constants/3(lambda1) -> [lambda1]
  [M] -> Product30/3
  Product16/1 -> Sum20/1
  [error_dot] -> Sign2/1, Abs1/1
  Sqrt1/1 -> Product16/1
  Sqrt/1 -> Product17/1
  Abs2/1 -> Sqrt2/1
  [lambda2] -> Sum26/1
  [zeta1] -> Product33/2
  Sign6/1 -> Product31/2
  [qd_ddot] -> Sum23/1
  [error_dot] -> Abs6/1
  [lambda2] -> Product32/1
  Constant3/1 -> Sum28/2, Sum/2
  [zeta1] -> Product11/1
  ANSFT Constants/1(xi1) -> [zeta1]
  [error] -> Sum18/2
  Abs7/1 -> Power5/1
  Sum17/1 -> [error]
  Power/1 -> Product11/2
  Constant2/1 -> Sum26/2
  ANSFT Constants/5(alpha) -> [alpha]
  [qd_dot] -> Sum19/1
  Product32/1 -> Divide3/2
  [pose_dot] -> Sum19/2
  Sum23/1 -> Product29/2
  Abs/1 -> Power/1
  Product33/1 -> Product34/1
  Product31/1 -> Divide3/1
  [error] -> Sign1/1, Abs/1
  Integrator14/1 -> Kt/1, [Kt]
  [Kt_dot] -> Kt_dot/1, Integrator14/1
  [Kt] -> Power2/1
  Product29/1 -> Bias/1
  Sum18/1 -> sigma/1, [sigma]
  Power1/1 -> Product12/2
  [qd] -> Sum17/1
  Abs6/1 -> Power4/1
  Sum26/1 -> Power4/2
  ANSFT Constants/2(xi2) -> [zeta2]
  Divide3/1 -> Product/1
  Sqrt2/1 -> Product16/2
  Product30/1 -> [fx]
  [lambda1] -> Product33/1
  Sign1/1 -> Product11/3
  qd/1 -> Bus Selector/1
  Bus Selector/2 -> [qd_dot]  "<qd_dot>"
  Bus Selector/1 -> [qd]  "<qd>"
  Bus Selector/3 -> [qd_ddot]  "<qd_ddot>"
  Reshape/1 -> Constants Functions/1(v)
  Constants Functions/1(Phi) -> Transpose/1  "phi"
  Constants Functions/2(M) -> [M]
  Rib function/1(Rbi) -> [Rbi]
  [v] -> Reshape/1
  Constants Functions/3(M_inv) -> [M_inv]
  [pose_g] -> Rib function/1(pose)
  Transpose/1 -> [Phi]  "phi_T"
  Mux28/1 -> [pose_g]
  [BF_dAtt] -> Selector18/1
  Mux29/1 -> [pose_dot], Matrix Multiply/2
  Selector18/1 -> Mux29/2
  Matrix Multiply/1 -> [v]
  [Rbi] -> Matrix Multiply/1
  [pos] -> Mux28/1
  Selector17/1 -> Mux28/2
  [BF_att] -> Selector17/1
  [vel] -> Mux29/1
  Bus Creator/1 -> u/1
  [error_dot] -> Bus Creator/3  "e_dot"
  [sigma] -> Bus Creator/5
  [Kt] -> Bus Creator/4  "kt"
  [F] -> Bus Creator/1  "u"
  [error] -> Bus Creator/2  "e"
  q/1 -> Bus Selector1/1
  Bus Selector1/1 -> [pos]  "<pos>"
  Bus Selector1/3 -> [BF_att]  "<bf_att>"
  Bus Selector1/2 -> [vel]  "<vel>"
  Bus Selector1/4 -> [BF_dAtt]  "<bf_datt>"
  Product34/1 -> Sum/1
  Sum/1 -> Product/2
  Bias/1 -> [u]  "u"
  [u] -> Matrix Multiply1/2
  [Rbi] -> Matrix Multiply1/1
  Matrix Multiply1/1 -> [F]
  [sigma] -> Product10/2
  Product10/1 -> Sum4/2
  [sigma] -> Abs4/1, Gain/1, Sign4/1
  Sqrt4/1 -> Product1/2
  Sqrt3/1 -> Product8/2
  [Kt] -> Gain3/1
  Gain3/1 -> Product1/1
  Sign3/1 -> Product8/3
  Gain2/1 -> Product10/1
  [sigma] -> Sign3/1, Abs3/1
  [Kt] -> Power3/1
  Sum4/1 -> Manual Variant Source3/1
  Abs3/1 -> Sqrt3/1
  Manual Variant Source3/1 -> Scope1/1, [u_aux]
  Product8/1 -> Sum4/1
  Sum1/1 -> Manual Variant Source3/2
  Power3/1 -> Gain2/1
  Gain1/1 -> Product8/1
  [epsilon] -> Product2/3
  Abs4/1 -> Sqrt4/1
  Sign4/1 -> Product1/3
  [Kt] -> Gain1/1
  Product1/1 -> Sum1/1
  [Kt] -> Product2/2
  Product2/1 -> Sum1/2
  Gain/1 -> Product2/1
  ANSFT Constants/7(epsilon) -> [epsilon]
  [error_dot] -> error_dot/1

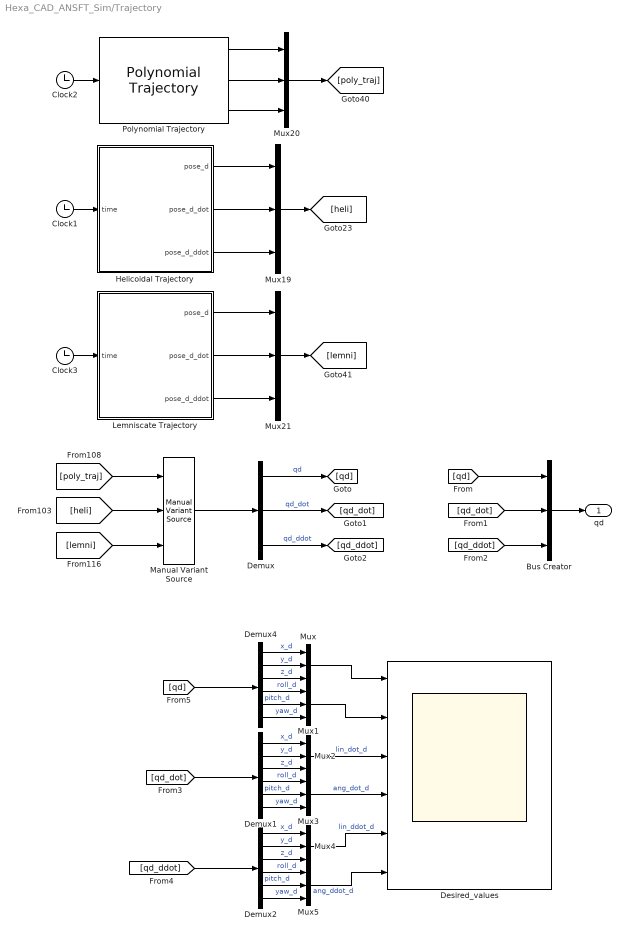
== system Hexa_CAD_ANSFT_Sim/Trajectory ==
  Bus Creator : BusCreator  Inputs=3
  Clock1 : Clock
  Clock2 : Clock
  Clock3 : Clock
  Demux : Demux  Outputs=3
  Demux1 : Demux  Outputs=6
  Demux2 : Demux  Outputs=6
  Demux4 : Demux  Outputs=6
  Desired_values : Scope  NumInputPorts=6
  Helicoidal Trajectory : MATLAB Function  TreatAsAtomicUnit=on
  Lemniscate Trajectory : MATLAB Function  TreatAsAtomicUnit=on
  Manual Variant Source : simulink/Signal Routing/Manual Variant Source  NumChoices=3  LabelModeActiveChoice=V_1
  Mux{,1..5,19..21} (9 alike) : Mux  Inputs=3
  Polynomial Trajectory : robotcorelib/Polynomial Trajectory  WaypointSource=Internal  Waypoints=zeros(6, 6)  TimePoints=[ 0, 12, 24, 36, 48, tf ]  TimeInterval=[ 1, 4 ]  Method=Cubic Polynomial  ParameterSource=Internal  VelocityBoundaryCondition=zeros( 6, 6 )  AccelerationBoundaryCondition=zeros( 2, 5 )  SimulateUsing=Interpreted execution
  qd : Outport
  wires:
  Polynomial Trajectory/2 -> Mux20/2
  Polynomial Trajectory/1 -> Mux20/1
  Lemniscate Trajectory/1(pose_d) -> Mux21/1
  Clock3/1 -> Lemniscate Trajectory/1(time)
  Polynomial Trajectory/3 -> Mux20/3
  Clock2/1 -> Polynomial Trajectory/1
  Helicoidal Trajectory/1(pose_d) -> Mux19/1
  Lemniscate Trajectory/3(pose_d_ddot) -> Mux21/3
  Mux21/1 -> [lemni]
  Mux19/1 -> [heli]
  Helicoidal Trajectory/2(pose_d_dot) -> Mux19/2
  Clock1/1 -> Helicoidal Trajectory/1(time)
  Mux20/1 -> [poly_traj]
  Helicoidal Trajectory/3(pose_d_ddot) -> Mux19/3
  Lemniscate Trajectory/2(pose_d_dot) -> Mux21/2
  Demux/3 -> [qd_ddot]  "qd_ddot"
  Demux/1 -> [qd]  "qd"
  Demux4/1 -> Mux/1  "x_d"
  Demux2/5 -> Mux5/2  "pitch_d"
  Demux/2 -> [qd_dot]  "qd_dot"
  [qd_ddot] -> Bus Creator/3
  Demux1/5 -> Mux3/2  "pitch_d"
  Demux1/3 -> Mux2/3  "z_d"
  Demux4/6 -> Mux1/3  "yaw_d"
  [qd_dot] -> Demux1/1
  [heli] -> Manual Variant Source/2
  Demux1/2 -> Mux2/2  "y_d"
  Mux1/1 -> Desired_values/2
  Demux4/3 -> Mux/3  "z_d"
  Demux4/2 -> Mux/2  "y_d"
  Demux1/1 -> Mux2/1  "x_d"
  [qd_ddot] -> Demux2/1
  Mux2/1 -> Desired_values/3  "lin_dot_d"
  Demux4/5 -> Mux1/2  "pitch_d"
  Mux5/1 -> Desired_values/6  "ang_ddot_d"
  Demux2/3 -> Mux4/3  "z_d"
  [qd] -> Demux4/1
  Mux3/1 -> Desired_values/4  "ang_dot_d"
  [qd_dot] -> Bus Creator/2
  Demux4/4 -> Mux1/1  "roll_d"
  Mux/1 -> Desired_values/1
  Demux1/4 -> Mux3/1  "roll_d"
  [lemni] -> Manual Variant Source/3
  Demux2/1 -> Mux4/1  "x_d"
  Demux1/6 -> Mux3/3  "yaw_d"
  Mux4/1 -> Desired_values/5  "lin_ddot_d"
  Bus Creator/1 -> qd/1
  Demux2/4 -> Mux5/1  "roll_d"
  [qd] -> Bus Creator/1
  [poly_traj] -> Manual Variant Source/1
  Manual Variant Source/1 -> Demux/1
  Demux2/6 -> Mux5/3  "yaw_d"
  Demux2/2 -> Mux4/2  "y_d"
